simulink model "Taller6_simulink"  (R2024a)
settings: Solver=VariableStepAuto  StartTime=0.0  StopTime=45  RelTol=1e-3
settings Model: Creator=UsuarioF  LastModifiedBy=UsuarioF

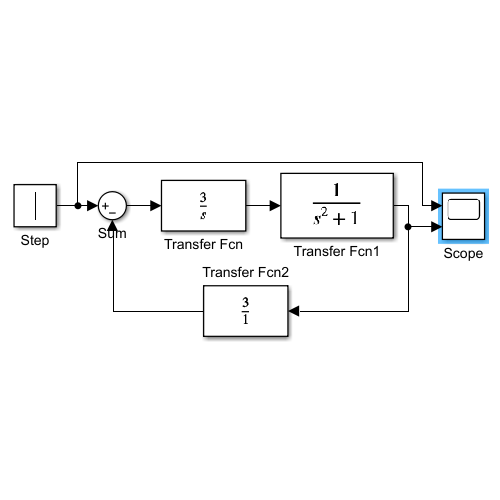
[thumbnail: Simulink's stored preview of the top-level diagram]
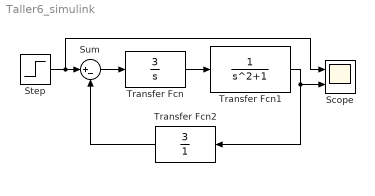
== system Taller6_simulink ==
  Scope : Scope  NumInputPorts=2
  Step : Step  SampleTime=0
  Sum : Sum  Inputs=|+-
  Transfer Fcn : TransferFcn  Numerator=[3]  Denominator=[1 0]
  Transfer Fcn1 : TransferFcn  Denominator=[1 0 1]
  Transfer Fcn2 : TransferFcn  Numerator=[3]  Denominator=[1]
  wires:
  Sum/1 -> Transfer Fcn/1
  Transfer Fcn/1 -> Transfer Fcn1/1
  Transfer Fcn1/1 -> Scope/2, Transfer Fcn2/1
  Step/1 -> Scope/1, Sum/1
  Transfer Fcn2/1 -> Sum/2
